simulink model "test_model_2018a"  (R2020a)
settings: Solver=VariableStepAuto  StartTime=0.0  StopTime=7  RelTol=1e-3
values from neighbouring files (symbols this model uses):
  A = sys_d.A    [discreteTest.m]    (also in discreteTestAttacked.m)
  B = sys_d.B    [discreteTest.m]    (also in discreteTestAttacked.m)
  C = sys_d.C    [discreteTest.m]    (also in discreteTestAttacked.m)
  D = sys_d.D    [discreteTest.m]    (also in discreteTestAttacked.m)
  K = [   5.261, -0.023 ... (first row only)    [discreteTest.m]    (also in discreteTestAttacked.m)
  steeringAngle = zeros(1, time)    [discreteTest.m]    (also in discreteTestAttacked.m)
  Ts = 0.04    [discreteTest.m]    (also in discreteTestAttacked.m)
undefined symbols (not defined in the file or in its folder): L
libraries: simulink x6
settings Model: Creator=Shreyash  LastModifiedBy=Shreyash
settings SolverCC: AlgebraicLoopSolver=LineSearch
settings DataIOCC: ReturnWorkspaceOutputs=off
settings DebuggingCC: ArithmeticOperatorsInVariantConditions=warning
settings SFSimCC: SimUseLocalCustomCode=off  CustomCodeUndefinedFunction=UseInterfaceOnly
settings RTWCC: RTWUseLocalCustomCode=off

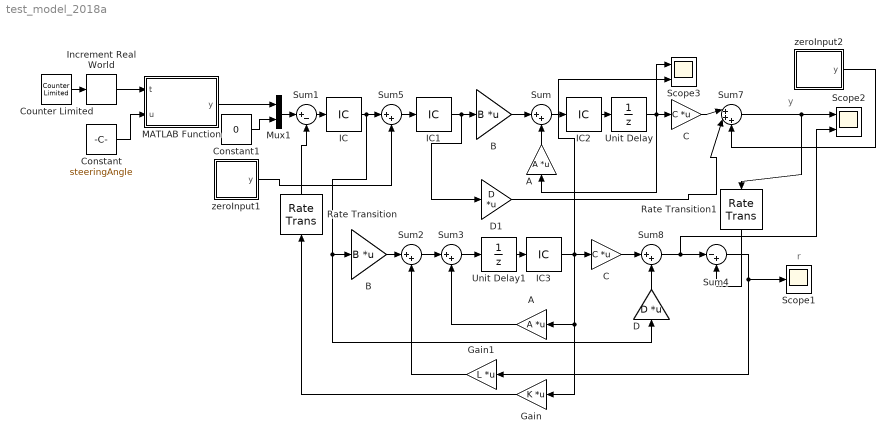
== system test_model_2018a ==
  note: y
  note: r
  A : Gain  Gain=A  Multiplication=Matrix(K*u)
  "A " : Gain  Gain=A  Multiplication=Matrix(K*u)
  B : Gain  Gain=B  Multiplication=Matrix(K*u)
  "B " : Gain  Gain=B  Multiplication=Matrix(K*u)
  C : Gain  Gain=C  Multiplication=Matrix(K*u)
  "C " : Gain  Gain=C  Multiplication=Matrix(K*u)
  Constant : Constant  Value=steeringAngle
  Constant1 : Constant  Value=0
  Counter Limited : simulink/Sources/Counter Limited  uplimit=124  tsamp=0.04
  D : Gain  Gain=D  Multiplication=Matrix(K*u)
  D1 : Gain  Gain=D  Multiplication=Matrix(K*u)
  Gain : Gain  Gain=K  Multiplication=Matrix(K*u)
  Gain1 : Gain  Gain=L  Multiplication=Matrix(K*u)
  IC{,1..3} (4 alike) : InitialCondition  Value=[0;0]
  Increment Real World : simulink/Additional Math & Discrete/Additional Math: Increment - Decrement/Increment Real World
      settings: SourceProductBaseCode=SL
  MATLAB Function : MATLAB Function  TreatAsAtomicUnit=on
  Mux1 : Mux  Inputs=2
  Rate Transition : RateTransition  InitialCondition=Ts  OutPortSampleTime=Ts
  Rate Transition1 : RateTransition  InitialCondition=Ts  OutPortSampleTimeMultiple=Ts  OutPortSampleTime=Ts
  Scope1 : Scope
  Scope2 : Scope  NumInputPorts=2
  Scope3 : Scope  NumInputPorts=2
  Sum{,2..3,5,8} (5 alike) : Sum  Inputs=|++
  Sum1 : Sum  Inputs=|+-
  Sum4 : Sum  Inputs=|-+
  Sum7 : Sum  Inputs=|+++
  Unit Delay : UnitDelay  SampleTime=-1  HasFrameUpgradeWarning=on
  Unit Delay1 : UnitDelay  SampleTime=-1  HasFrameUpgradeWarning=on
  zeroInput1 : Subsystem
  zeroInput2 : Subsystem
  wires:
  "B "/1 -> Sum/1
  Unit Delay/1 -> Scope3/1, "A "/1, "C "/1
  "A "/1 -> Sum/2
  Constant1/1 -> Mux1/2
  B/1 -> Sum2/1
  Sum2/1 -> Sum3/1
  Gain1/1 -> Sum2/2
  A/1 -> Sum3/2
  Sum4/1 -> Scope1/1, Gain1/1
  Rate Transition/1 -> Sum1/2
  Rate Transition1/1 -> Sum4/2
  Gain/1 -> Rate Transition/1
  Mux1/1 -> Sum1/1
  Counter Limited/1 -> Increment Real World/1
  Increment Real World/1 -> MATLAB Function/1(t)
  Constant/1 -> MATLAB Function/2(u)
  MATLAB Function/1(y) -> Mux1/1
  Sum5/1 -> IC1/1
  zeroInput1/1(y) -> Sum5/2
  IC1/1 -> D1/1, "B "/1
  IC/1 -> B/1, D/1, Sum5/1
  Sum1/1 -> IC/1
  Sum7/1 -> Rate Transition1/1, Scope2/1
  "C "/1 -> Sum7/1
  D1/1 -> Sum7/2
  C/1 -> Sum8/1
  Sum8/1 -> Sum4/1, Scope2/2
  D/1 -> Sum8/2
  Sum/1 -> IC2/1
  IC2/1 -> Unit Delay/1
  Sum3/1 -> Unit Delay1/1
  Unit Delay1/1 -> IC3/1
  IC3/1 -> Scope3/2, Gain/1, A/1, C/1
  zeroInput2/1(y) -> Sum7/3

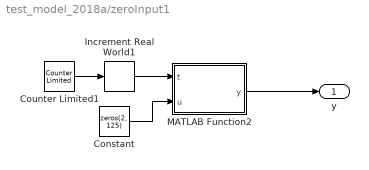
== system test_model_2018a/zeroInput1 ==
  Constant : Constant  Value=zeros(2, 125)
  Counter Limited1 : simulink/Sources/Counter Limited  uplimit=124  tsamp=0.04
  Increment Real World1 : simulink/Additional Math & Discrete/Additional Math: Increment - Decrement/Increment Real World
      settings: SourceProductBaseCode=SL
  MATLAB Function2 : MATLAB Function  TreatAsAtomicUnit=on
  y : Outport
  wires:
  Increment Real World1/1 -> MATLAB Function2/1(t)
  Counter Limited1/1 -> Increment Real World1/1
  Constant/1 -> MATLAB Function2/2(u)
  MATLAB Function2/1(y) -> y/1

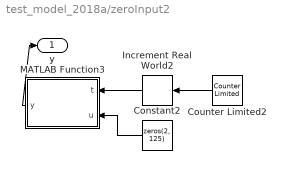
== system test_model_2018a/zeroInput2 ==
  Constant2 : Constant  Value=zeros(2, 125)
  Counter Limited2 : simulink/Sources/Counter Limited  uplimit=124  tsamp=0.04
  Increment Real World2 : simulink/Additional Math & Discrete/Additional Math: Increment - Decrement/Increment Real World
      settings: SourceProductBaseCode=SL
  MATLAB Function3 : MATLAB Function  TreatAsAtomicUnit=on
  y : Outport
  wires:
  Increment Real World2/1 -> MATLAB Function3/1(t)
  Counter Limited2/1 -> Increment Real World2/1
  Constant2/1 -> MATLAB Function3/2(u)
  MATLAB Function3/1(y) -> y/1

== matlab function test_model_2018a/MATLAB Function ==
  data: t input; u input; y output
function y = fcn(t, u)
y = u(t)*(pi/180)*0.0625;
end

== matlab function test_model_2018a/zeroInput2/MATLAB Function3 ==
  data: t input; u input; y output
function y = fcn(t, u)
y = u(:, t);
%for t = 1 :100
    %y = au(:, t);
    %y = (-1 + 2.*rand(1, 2))'; 
end

== matlab function test_model_2018a/zeroInput1/MATLAB Function2 ==
  data: t input; u input; y output
function y = fcn(t, u)
y = u(:, t);
%for t = 1 :100
    %y = au(:, t);
    %y = (-1 + 2.*rand(1, 2))'; 
end
